simulink model "RC_control"  (Simulink 6.6)
settings: Solver=FixedStepDiscrete  StartTime=0.0  StopTime=10.0  FixedStep=0.001  RelTol=1e-3
undefined symbols (not defined in the file): DiscIntNeverNeededParam, ecan1_init, ecan1_transmit_matlab, OC2max, u1
libraries: simulink x26, dsPICdrivers x11
(part 2 of 2)

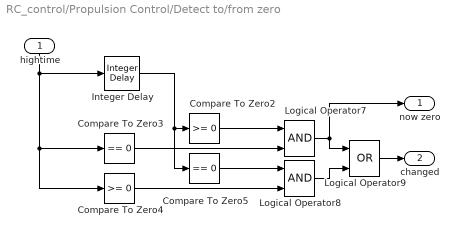
== system RC_control/Propulsion Control/Detect to/from zero ==
  hightime : Inport  Orientation=down
  Compare To Zero2 : simulink/Logic and Bit Operations/Compare To Zero  SystemSampleTime=-1  relop=>=  LogicOutDataTypeMode=boolean  ZeroCross=off
  Compare To Zero3 : simulink/Logic and Bit Operations/Compare To Zero  SystemSampleTime=-1  relop===  LogicOutDataTypeMode=boolean  ZeroCross=off
  Compare To Zero4 : simulink/Logic and Bit Operations/Compare To Zero  SystemSampleTime=-1  relop=>=  LogicOutDataTypeMode=boolean  ZeroCross=off
  Compare To Zero5 : simulink/Logic and Bit Operations/Compare To Zero  SystemSampleTime=-1  relop===  LogicOutDataTypeMode=boolean  ZeroCross=off
  Integer Delay : simulink/Discrete/Integer Delay  vinit=0.0  samptime=-1  NumDelays=1
  Logical Operator7 : Logic  AllPortsSameDT=off  OutDataTypeMode=Specify via dialog
  Logical Operator8 : Logic  AllPortsSameDT=off  OutDataTypeMode=Specify via dialog
  Logical Operator9 : Logic  Operator=OR  AllPortsSameDT=off  OutDataTypeMode=Specify via dialog
  now zero : Outport
  changed : Outport  Port=2
  wires:
  Logical Operator8/1 -> Logical Operator9/2
  Logical Operator7/1 -> Logical Operator9/1, now zero/1
  Compare To Zero4/1 -> Logical Operator8/2
  Compare To Zero5/1 -> Logical Operator8/1
  Compare To Zero3/1 -> Logical Operator7/2
  Compare To Zero2/1 -> Logical Operator7/1
  Integer Delay/1 -> Compare To Zero2/1, Compare To Zero5/1
  hightime/1 -> Integer Delay/1, Compare To Zero3/1, Compare To Zero4/1
  Logical Operator9/1 -> changed/1

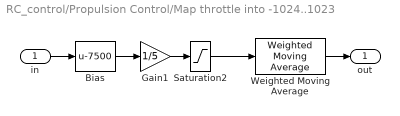
== system RC_control/Propulsion Control/Map throttle into -1024..1023 ==
  in : Inport
  Bias : Bias  Bias=-7500
  Gain1 : Gain  Gain=1/5
  Saturation2 : Saturate  UpperLimit=1023  LowerLimit=-1023
  Weighted Moving Average : simulink/Discrete/Weighted Moving Average  mgainval=[.3 .4 .3]  vinit=0.0  samptime=.01  GainDataType=uint(16)  MatRadixGroup=Best Precision: Matrix-wise  GainScaling=2^-10  OutDataType=sfix(16)  OutScaling=2^-10  DoSatur=off
  out : Outport
  wires:
  Bias/1 -> Gain1/1
  Gain1/1 -> Saturation2/1
  Saturation2/1 -> Weighted Moving Average/1
  in/1 -> Bias/1
  Weighted Moving Average/1 -> out/1

== system RC_control/Rudder Control/Map position  into -1024..1023 ==
  input : Inport
  Saturation : Saturate  UpperLimit=1023  LowerLimit=-1024
  Weighted Moving Average1 : simulink/Discrete/Weighted Moving Average  mgainval=[.5 .5]  vinit=0.0  samptime=-1  GainDataType=uint(16)  MatRadixGroup=Best Precision: Matrix-wise  GainScaling=2^-10  OutDataType=sfix(16)  OutScaling=2^-10  DoSatur=off
  mapped : Outport
  wires:
  Saturation/1 -> Weighted Moving Average1/1
  input/1 -> Saturation/1
  Weighted Moving Average1/1 -> mapped/1

== system RC_control/Rudder Control/Map rudder command into -1024..1023 ==
  input : Inport
  Bias1 : Bias  Bias=-941
  Gain4 : Gain  Gain=4
  Saturation3 : Saturate  UpperLimit=1023  LowerLimit=-1024
  Weighted Moving Average2 : simulink/Discrete/Weighted Moving Average  mgainval=[.3 .4 .3]  vinit=0.0  samptime=.01  GainDataType=uint(16)  MatRadixGroup=Best Precision: Matrix-wise  GainScaling=2^-10  OutDataType=sfix(16)  OutScaling=2^-10  DoSatur=off
  mapped : Outport
  wires:
  Saturation3/1 -> Weighted Moving Average2/1
  Gain4/1 -> Saturation3/1
  Bias1/1 -> Gain4/1
  input/1 -> Bias1/1
  Weighted Moving Average2/1 -> mapped/1

== matlab function Propulsion Control/Build CAN CC message/myMux ==
  data: u1 input inherited; y output inherited; u2 input inherited; u3 input inherited; u4 input inherited; u5 input inherited; u6 input inherited
function y = myMux(u1, u2, u3, u4, u5, u6)
y = [u1(1); u2(1); u3(1); u4(1); u5(1); u6(1);];

== matlab function Drive Motor Speed Message/myMux ==
  data: u1 input inherited; y output inherited; u2 input inherited; u3 input inherited; u4 input inherited; u5 input inherited
function y = myMux(u1, u2, u3, u4, u5)
u5_u16 = uint16(u5);
y = uint16([u1(1); u2(1); u3(1); u4(1); 0; 0; 0; 0;]);

len = length(u5);
if len > 1
    y(5) = bitor(bitshift(u5_u16(1),8),u5_u16(2));
elseif len > 0
    y(5) = u5_u16(1);
end
if len > 3
    y(6) = bitor(bitshift(u5_u16(3),8),u5_u16(4));
elseif len > 2
    y(6) = u5_u16(3);
end
if len > 5
    y(7) = bitor(bitshift(u5_u16(5),8),u5_u16(6));
elseif len > 4
    y(7) = u5_u16(5);
end
if len > 7
    y(8) = bitor(bitshift(u5_u16(7),8),u5_u16(8));
elseif len > 6
    y(8) = u5_u16(7);
end
